simulink model "dy"  (R2016a)
settings: Solver=VariableStepAuto  StartTime=0.0  StopTime=100  RelTol=1e-3
libraries: simulink x1
settings Model: Creator=asus  LastModifiedBy=asus

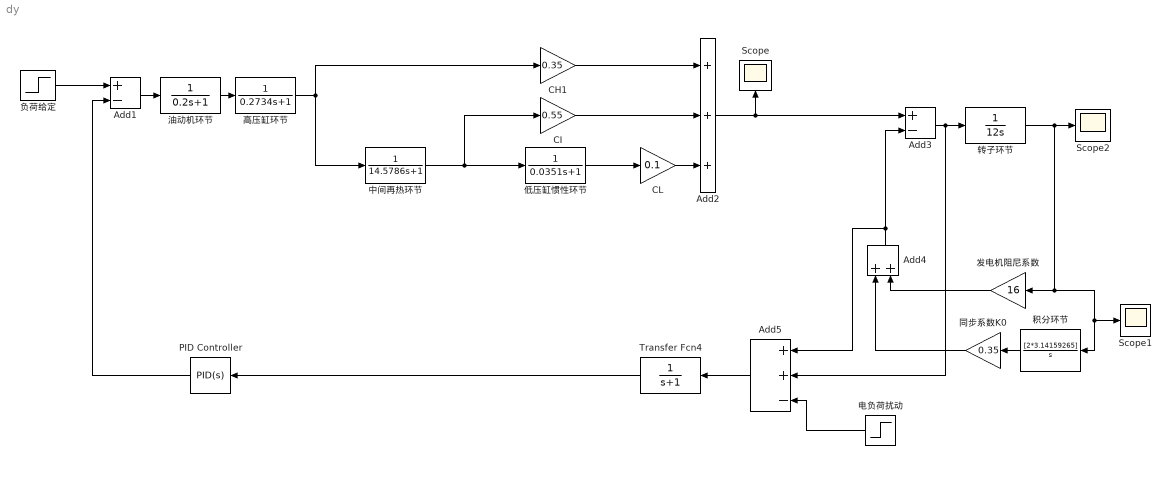
== system dy ==
  Add1 : Sum  Inputs=+-
  Add2 : Sum  Inputs=+++
  Add3 : Sum  Inputs=+-
  Add4 : Sum
  Add5 : Sum  Inputs=++-
  CH1 : Gain  Gain=0.35
  CI : Gain  Gain=0.55
  CL : Gain  Gain=0.1
  PID Controller : simulink/Continuous/PID Controller  Controller=PID  TimeDomain=Continuous-time  SampleTime=-1  IntegratorMethod=Forward Euler  FilterMethod=Forward Euler  Form=Parallel  UseFilter=on  ControllerParametersSource=internal  P=1  I=1  D=0  N=100  InitialConditionSource=internal  InitialConditionForIntegrator=0  InitialConditionForFilter=0  ExternalReset=none  LimitOutput=off  UpperSaturationLimit=inf  LowerSaturationLimit=-inf  LinearizeAsGain=on  AntiWindupMode=none  Kb=1  TrackingMode=off  Kt=1  PParamMin=[]  PParamMax=[]  IParamMin=[]  IParamMax=[]  DParamMin=[]  DParamMax=[]  NParamMin=[]  NParamMax=[]  KbParamMin=[]  KbParamMax=[]  KtParamMin=[]  KtParamMax=[]  POutMin=[]  POutMax=[]  IOutMin=[]  IOutMax=[]  DOutMin=[]  DOutMax=[]  NOutMin=[]  NOutMax=[]  KbOutMin=[]  KbOutMax=[]  KtOutMin=[]  KtOutMax=[]  IntegratorOutMin=[]  IntegratorOutMax=[]  FilterOutMin=[]  FilterOutMax=[]  SumOutMin=[]  SumOutMax=[]  SumI1OutMin=[]  SumI1OutMax=[]  SumI2OutMin=[]  SumI2OutMax=[]  SumI3OutMin=[]  SumI3OutMax=[]  SumDOutMin=[]  SumDOutMax=[]  SaturationOutMin=[]  SaturationOutMax=[]  IntegratorContinuousStateAttributes=''  IntegratorStateMustResolveToSignalObject=off  IntegratorRTWStateStorageClass=Auto  FilterContinuousStateAttributes=''  FilterStateMustResolveToSignalObject=off  FilterRTWStateStorageClass=Auto  DifferentiatorICPrevScaledInput=0  DifferentiatorOutMin=[]  DifferentiatorOutMax=[]
  Scope : Scope
  Scope1 : Scope
  Scope2 : Scope
  Transfer Fcn4 : TransferFcn  Denominator=[1 1]
  中间再热环节 : TransferFcn  Denominator=[14.5786 1]
  低压缸惯性环节 : TransferFcn  Denominator=[0.0351 1]
  发电机阻尼系数 : Gain  Gain=16
  同步系数K0 : Gain  Gain=0.35
  油动机环节 : TransferFcn  Denominator=[0.2 1]
  电负荷扰动 : Step  Time=0  Before=0.5  After=0  SampleTime=0.1
  积分环节 : TransferFcn  Numerator=[2*3.14159265]  Denominator=[1 0]
  负荷给定 : Step  Time=10  After=0.5  SampleTime=0.01
  转子环节 : TransferFcn  Denominator=[12 0]
  高压缸环节 : TransferFcn  Denominator=[0.2734 1]
  wires:
  负荷给定/1 -> Add1/1
  Add1/1 -> 油动机环节/1
  油动机环节/1 -> 高压缸环节/1
  高压缸环节/1 -> CH1/1, 中间再热环节/1
  中间再热环节/1 -> CI/1, 低压缸惯性环节/1
  低压缸惯性环节/1 -> CL/1
  CL/1 -> Add2/3
  CI/1 -> Add2/2
  CH1/1 -> Add2/1
  Add2/1 -> Add3/1, Scope/1
  Add3/1 -> 转子环节/1, Add5/2
  Add4/1 -> Add3/2, Add5/1
  发电机阻尼系数/1 -> Add4/2
  转子环节/1 -> 积分环节/1, Scope1/1, 发电机阻尼系数/1, Scope2/1
  积分环节/1 -> 同步系数K0/1
  同步系数K0/1 -> Add4/1
  电负荷扰动/1 -> Add5/3
  Add5/1 -> Transfer Fcn4/1
  Transfer Fcn4/1 -> PID Controller/1
  PID Controller/1 -> Add1/2
